simulink model "anti_aliasing_test"  (R2014b)
settings: Solver=ode45  StartTime=0.0  StopTime=20.0  RelTol=1e-3
values from neighbouring files (symbols this model uses):
  h = 2/10    (= 0.2)    [aliasing_example_model.m]    (also in notch_filter_example.m = 0.5; notch_filter_tustin_example.m = 0.5; sixty_hertz_hum_alias.m = 0.1)
libraries: dsparch4 x2
settings Model: Creator=kjartan  LastModifiedBy=kjartan

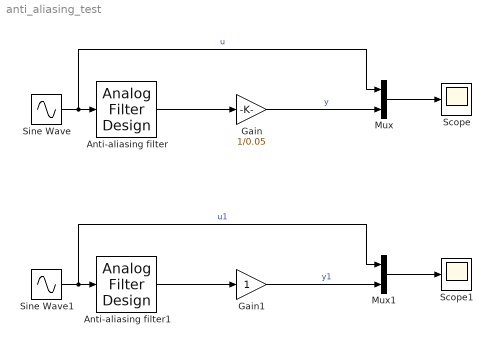
== system anti_aliasing_test ==
  Anti-aliasing filter : dsparch4/Analog Filter Design  method=Bessel  filttype=Lowpass  N=4  Wlo=1.67*0.3*pi/h  Whi=80  Rp=2  Rs=40
  Anti-aliasing filter1 : dsparch4/Analog Filter Design  method=Bessel  filttype=Lowpass  N=4  Wlo=1.67*0.3*pi/h  Whi=80  Rp=2  Rs=40
  Gain : Gain  Gain=1/0.05
  Gain1 : Gain
  Mux : Mux  Inputs=2
  Mux1 : Mux  Inputs=2
  Scope : Scope
      settings: ShowLegends=on
  Scope1 : Scope
      settings: ShowLegends=on
  Sine Wave : Sin  Frequency=pi/h  SampleTime=0
  Sine Wave1 : Sin  Frequency=pi/h/10  SampleTime=0
  wires:
  Sine Wave/1 -> Mux/1, Anti-aliasing filter/1  "u"
  Anti-aliasing filter/1 -> Gain/1
  Gain/1 -> Mux/2  "y"
  Mux/1 -> Scope/1
  Sine Wave1/1 -> Mux1/1, Anti-aliasing filter1/1  "u1"
  Anti-aliasing filter1/1 -> Gain1/1
  Gain1/1 -> Mux1/2  "y1"
  Mux1/1 -> Scope1/1
